simulink model "p6"  (R2016a)
settings: Solver=FixedStepDiscrete  StartTime=0.0  StopTime=10.0  RelTol=1e-3
libraries: dspvision x1, dspobslib x1
settings Model: Creator=sebi_  LastModifiedBy=adrian.amariei
settings DataIOCC: LimitDataPoints=on
settings DebuggingCC: AllowSymbolicDim=off
settings ModelReferenceCC: PropagateSignalLabelsOutOfModel=off
settings GRTTargetCC: GeneratePreprocessorConditionals=Use local settings

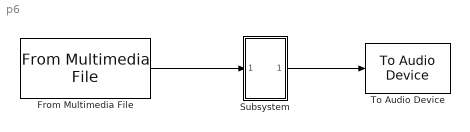
== system p6 ==
  From Multimedia File : dspvision/From Multimedia File  inputFilename=C:\Users\adrian.amariei\Desktop\dsptest\Kalimba.mp3  loop=on  numPlays=inf  outputStreams=Audio only  videoDataType=single  audioDataType=double  inheritSampleTime=on  userDefinedSampleTime=1/30  noAudioOutput=off  isIntensityVideo=off  fourcc=RGB  colorVideoFormat=Separate color signals  outputEOF=off  dataOrg=Column-major  audioFrameSize=1  computeAudioFrameSize=off  outSamplingMode=Sample based
  Subsystem : Subsystem
  To Audio Device : dspobslib/To Audio Device  deviceName=Default  inheritSampleRate=on  sampleRate=44100  deviceDatatype=Determine from input data type  autoBufferSize=on  bufferSize=4096  queueDuration=1.0  defaultOutputChannelMapping=on  outputChannelMapping=1:2  outputNumUnderrunSamples=off
  wires:
  From Multimedia File/1 -> Subsystem/1(In1)
  Subsystem/1(Out1) -> To Audio Device/1

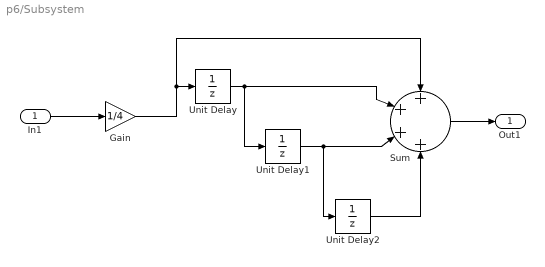
== system p6/Subsystem ==
  In1 : Inport
  Gain : Gain  Gain=1/4
  Sum : Sum  Inputs=++++
  Unit Delay : UnitDelay  SampleTime=-1
  Unit Delay1 : UnitDelay  SampleTime=-1
  Unit Delay2 : UnitDelay  SampleTime=-1
  Out1 : Outport
  wires:
  Sum/1 -> Out1/1
  In1/1 -> Gain/1
  Gain/1 -> Sum/1, Unit Delay/1
  Unit Delay/1 -> Unit Delay1/1, Sum/2
  Unit Delay1/1 -> Unit Delay2/1, Sum/3
  Unit Delay2/1 -> Sum/4
